simulink model "Model_FC_v16_Edit_for_Full_Scale_Fuel_Cell_GAS"  (R2018a)
settings: Solver=VariableStepAuto  StartTime=0  StopTime=inf  FixedStep=0.01  RelTol=1e-3  EnableMultiTasking=on
undefined symbols (not defined in the file): sigbuilder_block
libraries: fl_lib x8, simulink x6, nesl_utility x4, autolibdcdc x1, powerlib x1
(part 1 of 3)
settings Model: SimulationMode=accelerator  Creator=Mina  LastModifiedBy=Mina
settings SolverCC: ZeroCrossControl=EnableAll  ZeroCrossAlgorithm=Adaptive
settings DataIOCC: LimitDataPoints=on  SaveFormat=Array
settings OptimizationCC: BlockReduction=off  ConditionallyExecuteInputs=off  EfficientMapNaN2IntZero=off  LifeSpan=inf  SimCompilerOptimization=on  AccelVerboseBuild=on
settings DebuggingCC: IgnoredZcDiagnostic=none  SFUnexpectedBacktrackingDiag=warning  SFNoUnconditionalDefaultTransitionDiag=warning  SFExecutionAtInitializationDiag=none
settings HardwareCC: ProdBitPerPointer=32  ProdBitPerSizeT=32  ProdBitPerPtrDiffT=32  ProdLargestAtomicFloat=None  ProdIntDivRoundTo=Undefined  ProdEndianess=Unspecified  ProdWordSize=32  ProdHWDeviceType=32-bit Generic  TargetBitPerPointer=64  TargetBitPerSizeT=64  TargetBitPerPtrDiffT=64  TargetLongLongMode=on  TargetIntDivRoundTo=Zero  TargetEndianess=LittleEndian  TargetWordSize=64  TargetHWDeviceType=MATLAB Host  ProdEqTarget=off
settings ModelReferenceCC: PropagateSignalLabelsOutOfModel=off
settings CodeAppCC: MaxIdLength=128  StateflowObjectComments=on
settings GRTTargetCC: TargetLangStandard=C89/C90 (ANSI)  CombineOutputUpdateFcns=off  GRTInterface=on
settings ConfigComp: CovMetricSettings=dw  CovHtmlReporting=on  CovSaveCumulativeToWorkspaceVar=on  CovSaveSingleToWorkspaceVar=on  CovExternalEMLEnable=off
settings SimscapeCC: SimscapeNormalizeSystem=off

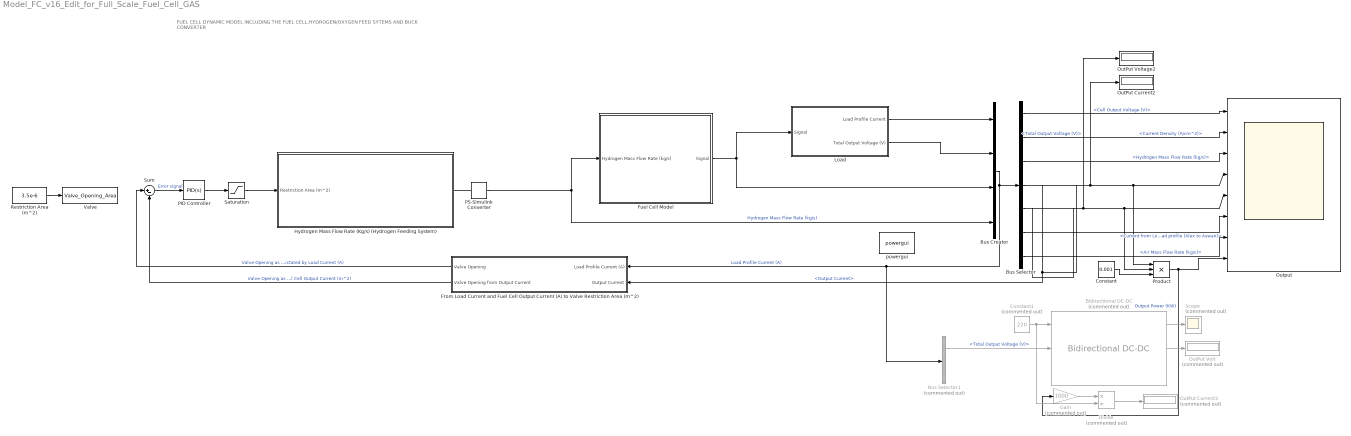
== system Model_FC_v16_Edit_for_Full_Scale_Fuel_Cell_GAS ==
  note: FUEL CELL DYNAMIC MODEL INCLUDING THE FUEL CELL,HYDROGEN/OXYGEN FEED SYTEMS AND BUCK CONVERTER
  Bidirectional DC-DC : autolibdcdc/Bidirectional DC-DC  Commented=on  Tc=1/1000  Vinit=0  Plimit=100000  param_loss=Single efficiency measurement  eff=98  v_loss_bp=[0 200 400 600 800 1000]  i_loss_bp=[0 25 50 75 100]  losses_table=[100 100 100 100 100;100 150 200 250 300;100 200 300 400 500;100 250 400 550 700;100 300 500 700 900;100 350 600 850 1100]  v_eff_bp=[200 400 600 800 1000]  i_eff_bp=[25 50 75 100]  efficiency_table=[96.2 98.1 98.7 99;98.1 99 99.4 99.5;98.7 99.4 99.6 99.7;99 99.5 99.7 99.8;99.2 99.6 99.7 99.8]  x_v_bp=[-1000 -800 -600 -400 -200 200 400 600 800 1000]  x_i_bp=[-100 -75 -50 -25 25 50 75 100]  x_losses_mat=[200.400801603196 225.67703109328 200.803212851408 201.612903225806 199.999999999997 200 225 200;160.320641282556 180.541624874624 201.005025125625 202.020202020203 200 200 180 160;180.541624874624 180.722891566267 181.086519114686 197.568389057748 194.999999999999 179.999999999997 180 180;201.005025125625 181.086519114686 202.020202020203 193.67991845056 190 200 179.999999999997 200;202.020202020203 197.568389057748 193.67991845056 197.505197505197 190 190 194.999999999999 200;200 194.999999999999 190 190 197.505197505197 193.67991845056 197.568389057748 202.020202020203;200 179.999999999997 200 190 193.67991845056 202.020202020203 181.086519114686 201.005025125625;180 180 179.999999999997 194.999999999999 197.568389057748 181.086519114686 180.722891566267 180.541624874624;160 180 200 200 202.020202020203 201.005025125625 180.541624874624 160.320641282556;200 225 200 199.999999999997 201.612903225806 200.803212851408 225.67703109328 200.400801603196]
      settings: SourceProductName=Powertrain Blockset  SourceProductBaseCode=PW
  Bus Creator : BusCreator  Inputs=4
  Bus Selector : BusSelector  OutputSignals=signal3.Cell Output Voltage (V),signal3.Current Density (A/cm^2),Hydrogen Mass Flow Rate (kg/s),signal3.Output Current,Total Output Voltage (V),Current from Load profile (Alex to Aswan),signal3.Air Mass Flow Rate (kg/s)
  Bus Selector1 : BusSelector  Commented=on  OutputSignals=Total Output Voltage (V),signal3.Output Current
  Constant : Constant  Value=0.001
  Constant1 : Constant  Commented=on  Value=220
  Divide : Product  Commented=on  Inputs=*/
  From Load Current and Fuel Cell Output Current (A) to Valve Restriction Area (m^2) : Subsystem
  Fuel Cell Model : Subsystem  mask(Fuel Cell Model){Temperature_c=80, Hydrogen_Pressure_atm=8, Air_Pressure_atm=8, Number_of_cells=208, Cell_Area_cm_squared=4397.14, Alpha_charge_Transfer_Coefficient=0.5, Exchange_Current_Density_i0=0.00000012246, Internal_Resistance_r=0.019, Amplification_Constant_Alpha1=0.085, Limiting_Current_Density_i_l=2, Mass_Transport_Limit_k=1.1, Dynamic_Response=[5 1]}
      mask prompts: Temperature_c "Temperature (c)"; Hydrogen_Pressure_atm "Hydrogen Pressure (atm)"; Air_Pressure_atm "Air Pressure (atm)"; Number_of_cells "Number Of Cells"; Cell_Area_cm_squared "Cell Area (cm^2)"; Alpha_charge_Transfer_Coefficient "Alpha (Charge Transfer Coefficient)"; Exchange_Current_Density_i0 "Exchange Current Density (i_0)(A/cm^2)"; Internal_Resistance_r "Internal Resistance (r)(Ohm)"; Amplification_Constant_Alpha1 "Amplification Constant (Alpha1)"; Limiting_Current_Density_i_l "Limiting Current Density (i_L)(A/cm^2)"; Mass_Transport_Limit_k "Mass Transport Limit (k)"; Dynamic_Response "Cell Dynamic Response (s)"
      mask help:
      | This is a mathematical Fuel Cell dynamic model. It operates under the Following Assumptions:
      | 1-The model is dynamic ,ie, it models the fuel cell behavior with respect to time.
      | 2-Fuel Cell Temperature is Constant.
      | 3-No Excess Hydrogen ,ie, Every Hydrogen molecule that enters the fuel cell Stack reacts to produce electricity.
      | 4-No excess Air.
      | 5-Concentration Losses are not calculated in the Model as we will never approach this region during operation.
      mask TypeOptions Temperature_c:
      | Stack Temperature
      | (C)/Value
      mask TypeOptions Hydrogen_Pressure_atm: Hydrogen Pressure (atm)/Value
      mask TypeOptions Air_Pressure_atm: Air Pressue (atm)/Value
      mask TypeOptions Number_of_cells: Number of Cells/Value
      mask TypeOptions Cell_Area_cm_squared:
      | Cell Area
      | (cm^2)/Value
      mask TypeOptions Alpha_charge_Transfer_Coefficient:
      | From Current Density (A//cm^2)
      | To
      | Overvoltages (V)/Activation Overvoltage/Alpha
      | Charge Transfer Coefficient1/Value
      mask TypeOptions Exchange_Current_Density_i0:
      | From Current Density (A//cm^2)
      | To
      | Overvoltages (V)/Activation Overvoltage/Reference Exchange Current Density
      | (I_0)1/Value
      mask TypeOptions Internal_Resistance_r:
      | From Current Density (A//cm^2)
      | To
      | Overvoltages (V)/Ohmic Overvoltage/Internal Resistance
      | (r)/Value
      mask TypeOptions Amplification_Constant_Alpha1:
      | From Current Density (A//cm^2)
      | To
      | Overvoltages (V)/Concentration Overvoltage/Amplification Constant
      | Alpha2/Value
      mask TypeOptions Limiting_Current_Density_i_l:
      | From Current Density (A//cm^2)
      | To
      | Overvoltages (V)/Concentration Overvoltage/Limiting Current
      | (i_L)1/Value
      mask TypeOptions Mass_Transport_Limit_k:
      | From Current Density (A//cm^2)
      | To
      | Overvoltages (V)/Concentration Overvoltage/Mass Transport Constant
      | (K)1/Value
      mask TypeOptions Dynamic_Response: Cell dynamic/Denominator
      mask DialogControl Operating_Conditions Prompt: Operating Conditions
      mask DialogControl Fuel_Cell_Parameters Prompt: Fuel Cell Parameters
      mask Display: image(imread('power_fuelcell.png'));port_label('output',1,'m');
  Gain : Gain  Commented=on  Gain=1000
  Hydrogen Mass Flow Rate (Kg/s) (Hydrogen Feeding System) : Subsystem
  Load : Subsystem
  OutPut Current2 : Display
  OutPut Current3 : Display  Commented=on
  OutPut Volt : Display  Commented=on
  OutPut Voltage2 : Display
  "Output " : Scope  NumInputPorts=8
  PID Controller : simulink/Continuous/PID Controller  Controller=PID  TimeDomain=Continuous-time  SampleTime=-1  IntegratorMethod=Forward Euler  FilterMethod=Forward Euler  Form=Parallel  UseFilter=on  ControllerParametersSource=internal  P=0.5  I=0.7  D=0.01  N=100  InitialConditionSource=internal  InitialConditionForIntegrator=0  InitialConditionForFilter=0  ExternalReset=none  LimitOutput=on  UpperSaturationLimit=1.5e-5  LowerSaturationLimit=-inf  LinearizeAsGain=on  AntiWindupMode=none  Kb=1  TrackingMode=off  Kt=1  PParamMin=[]  PParamMax=[]  IParamMin=[]  IParamMax=[]  DParamMin=[]  DParamMax=[]  NParamMin=[]  NParamMax=[]  KbParamMin=[]  KbParamMax=[]  KtParamMin=[]  KtParamMax=[]  POutMin=[]  POutMax=[]  IOutMin=[]  IOutMax=[]  DOutMin=[]  DOutMax=[]  NOutMin=[]  NOutMax=[]  KbOutMin=[]  KbOutMax=[]  KtOutMin=[]  KtOutMax=[]  IntegratorOutMin=[]  IntegratorOutMax=[]  FilterOutMin=[]  FilterOutMax=[]  SumOutMin=[]  SumOutMax=[]  SumI1OutMin=[]  SumI1OutMax=[]  SumI2OutMin=[]  SumI2OutMax=[]  SumI3OutMin=[]  SumI3OutMax=[]  SumDOutMin=[]  SumDOutMax=[]  SaturationOutMin=[]  SaturationOutMax=[]  IntegratorContinuousStateAttributes=''  IntegratorStateMustResolveToSignalObject=off  IntegratorRTWStateStorageClass=Auto  FilterContinuousStateAttributes=''  FilterStateMustResolveToSignalObject=off  FilterRTWStateStorageClass=Auto  DifferentiatorICPrevScaledInput=0  DifferentiatorOutMin=[]  DifferentiatorOutMax=[]  InitialConditionSetting=State (most efficient)  FilterDiffOutCoefMin=[]  FilterDiffOutCoefMax=[]  SumDenOutMin=[]  SumDenOutMax=[]  SumNumOutMin=[]  SumNumOutMax=[]  ReciprocalOutMin=[]  ReciprocalOutMax=[]  DivideOutMin=[]  DivideOutMax=[]  TunerSelectOption=Transfer Function Based (PID Tuner App)
  PS-Simulink Converter : nesl_utility/PS-Simulink Converter  PhysicalDomain=network_engine_domain  SubClassName=ps_output  LeftPortType=input  RightPortType=output  PseudoPeriodic=off  Frequencies=[]  Unit=1  AffineConversion=off
  Product : Product  Inputs=3
  "Restriction Area (m^2) " : Constant  Value=3.5e-6  VectorParams1D=off
  Saturation : Saturate  UpperLimit=2.7e-5  LowerLimit=0
  Scope : Scope  Commented=on
  Sum : Sum  Inputs=|+-
  Valve : ToWorkspace  VariableName=Valve_Opening_Area  SaveFormat=Timeseries  SampleTime=-1
  powergui : powerlib/powergui  Priority=1  SimulationMode=Discrete  SampleTime=50e-6  frequency=60  Iterations=50  frequencyindice=0  Pbase=100e6  ErrMax=1e-4  UnitsV=kV  UnitsW=MW  buscounter=0  FunctionMessages=off  echomessages=off  EnableUseOfTLC=off  CurrentSourceSwitches=off  DisableSnubberDevices=off  DisableRonSwitches=off  DisableVfSwitches=off  DisplayEquations=off  SolverType=Tustin/Backward Euler (TBE)  Interpol=off  ExternalGateDelay=off  methode=off  Ts=100  x0status=blocks  SPID=off  SwTol=0  HookPort=off  RestoreLinks=warning  ResistiveCurrentMeasurement=off  Frange=[0:2:500]  Ylog=off  Xlog=on  ShowGrid=off  save=off  variable=ZData  structure=0  ZoomFFT=off  StartTime=0.0  cycles=1  DisplayStyle=1  fundamental=60  FreqAxis=off  MaxFrequency=1000  frequencyindicesteady=1  RmsSteady=1  display=off
  wires:
  Fuel Cell Model/1(Signal) -> Bus Creator/3, Load/1(Signal)
  PS-Simulink Converter/1 -> Fuel Cell Model/1(Hydrogen Mass Flow Rate (kg/s)), Bus Creator/4  "Hydrogen Mass Flow Rate (kg/s)"
  Load/1(Load Profile Current) -> Bus Creator/1
  Load/2(Total Output Voltage (V)) -> Bus Creator/2
  Bus Selector/1 -> "Output "/1  "<Cell Output Voltage (V)>"
  Bus Selector/2 -> "Output "/2  "<Current Density (A/cm^2)>"
  Bus Selector/3 -> "Output "/3  "<Hydrogen Mass Flow Rate (kg/s)>"
  Bus Selector/4 -> OutPut Current2/1, Product/1, "Output "/4, From Load Current and Fuel Cell Output Current (A) to Valve Restriction Area (m^2)/2(Output Current)  "<Output Current>"
  Bus Selector/5 -> OutPut Voltage2/1, Product/2, "Output "/5  "<Total Output Voltage (V)>"
  From Load Current and Fuel Cell Output Current (A) to Valve Restriction Area (m^2)/1(Valve Opening) -> Sum/1  "Valve Opening as dictated by Load Current (A)"
  "Restriction Area (m^2) "/1 -> Valve/1
  From Load Current and Fuel Cell Output Current (A) to Valve Restriction Area (m^2)/2(Valve Opening from Output Current) -> Sum/2  "Valve Opening as dictated by Fuel Cell Output Current (m^2)"
  Sum/1 -> PID Controller/1  "Error signal"
  Bus Creator/1 -> From Load Current and Fuel Cell Output Current (A) to Valve Restriction Area (m^2)/1(Load Profile Current (A)), Bus Selector1/1, Bus Selector/1  "Load Profile Current (A)"
  Bus Selector/6 -> "Output "/6  "<Current from Load profile (Alex to Aswan)>"
  PID Controller/1 -> Saturation/1
  Saturation/1 -> Hydrogen Mass Flow Rate (Kg/s) (Hydrogen Feeding System)/1(Restriction Area (m^2))
  Bus Selector/7 -> "Output "/7  "<Air Mass Flow Rate (kg/s)>"
  Product/1 -> Gain/1, "Output "/8  "Output Power (KW)"
  Constant/1 -> Product/3
  Constant1/1 -> Divide/2, Bidirectional DC-DC/1
  Bidirectional DC-DC/1 -> Scope/1
  Bidirectional DC-DC/2 -> OutPut Volt/1
  Bus Selector1/1 -> Bidirectional DC-DC/2  "<Total Output Voltage (V)>"
  Divide/1 -> OutPut Current3/1
  Gain/1 -> Divide/1
  connections:
  PS-Simulink Converter/LConn1 -- Hydrogen Mass Flow Rate (Kg/s) (Hydrogen Feeding System)/RConn1

== system Model_FC_v16_Edit_for_Full_Scale_Fuel_Cell_GAS/From Load Current and Fuel Cell Output Current (A) to Valve Restriction Area (m^2) ==
  note: (3.0735e-14*(u(1)^3)) + (-5.0428e-11*(u(1)^2)) +(4.1772e-08*u(1)) + 2.7105e-07
  note: FEEDBACK BLOCK
  note: This block is the feedback block that controls the Flow control valve of the Hydrogen feeding system
      | I NPUTS: A) load Current (A) OUTPUTS: A) valve Restriction Area(m^2) as dictated by the Load Current
      | B) Output Current of the Fuel Cell (A) B) valve Restriction Area (m^2) as dictated by the Fuel Cell output current
  Load Profile Current (A) : Inport
  Output Current : Inport  Port=2
  Subsystem : Subsystem
  Subsystem1 : Subsystem
  Valve Opening : Outport
  Valve Opening from Output Current : Outport  Port=2
  wires:
  Output Current/1 -> Subsystem/1(In1)
  Subsystem/1(Valve Opening from Output Current) -> Valve Opening from Output Current/1
  Load Profile Current (A)/1 -> Subsystem1/1(In1)
  Subsystem1/1(Out1) -> Valve Opening/1

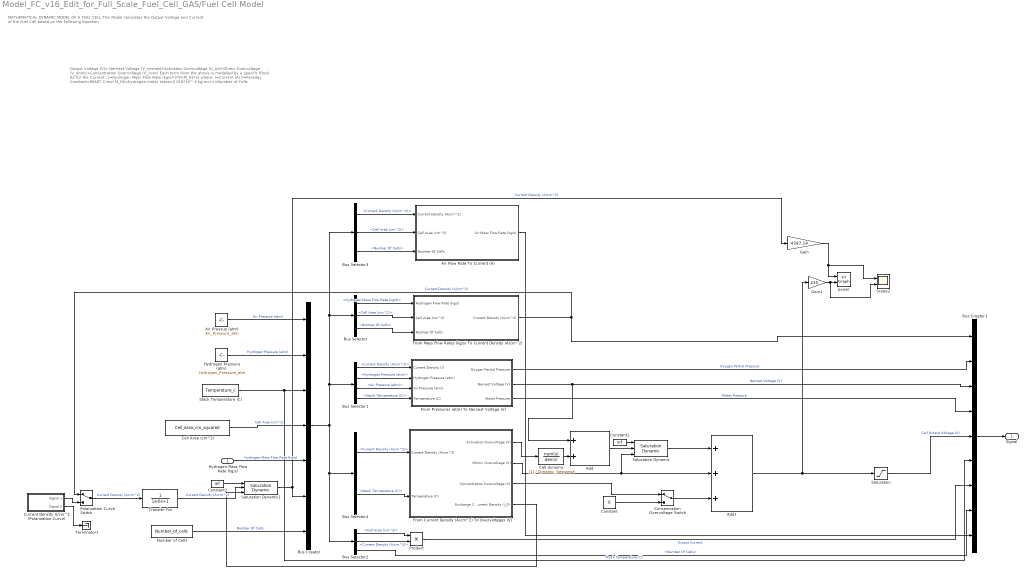
== system Model_FC_v16_Edit_for_Full_Scale_Fuel_Cell_GAS/Fuel Cell Model ==
  note: Output Voltage (V)= Nernest Voltage (V_nernest)-Activation Overvoltage (V_Act)-Ohmic Overvoltage (V_ohmic)-Concentration Overvoltage (V_conc)
      | Each term from the above is modelled by a specific Block.
      | As for the Current :
      |
      | I=Hydrogen Mass Flow Rate (kg/s)*2*F/(M_H2*n)
      | where: I=Current (A)
      | F=Faraday Constant=96487 C/mol
      | M_H2=hydrogen molar mass=2.016*10^-3 kg/mol
      | n=Number of Cells
  note: MATHEMATICAL DYNAMIC MODEL OF A FUEL CELL
      | This Model calculates the Output Voltage and Current of the Fuel Cell based on the Following Equation
  Hydrogen Mass Flow Rate (kg/s) : Inport
  " From Current Density (A/cm^2) To Overvoltages (V)" : Subsystem
  Add : Sum
  Add1 : Sum  Inputs=+++
  Air Flow Rate To Current (A) : Subsystem
  Air Pressue (atm) : Constant  Value=Air_Pressure_atm
  Bus Creator : BusCreator  Inputs=7
  Bus Creator1 : BusCreator  Inputs=9
  Bus Selector : BusSelector  OutputSignals=Hydrogen Mass Flow Rate (kg/s),Cell Area (cm^2),Number Of Cells
  Bus Selector1 : BusSelector  OutputSignals=Current Density (A/cm^2),Hydrogen Pressure (atm),Air Pressure (atm),Stack Temperature (C)
  Bus Selector2 : BusSelector  OutputSignals=Cell Area (cm^2),Current Density (A/cm^2),Number Of Cells
  Bus Selector3 : BusSelector  OutputSignals=Current Density (A/cm^2),Cell Area (cm^2),Number Of Cells
  Bus Selector4 : BusSelector  OutputSignals=Current Density (A/cm^2),Stack Temperature (C)
  Cell Area (cm^2) : Constant  Value=Cell_Area_cm_squared
  Cell dynamic : TransferFcn  Denominator=Dynamic_Response
  Concentration Overvoltage Switch : ManualSwitch
  Constant : Constant  Value=0
  Constant1 : Constant  Value=inf
  Constant2 : Constant  Value=inf
  Current Density A/cm^2 (Polarization Curve) : Subsystem  Tag=STV Subsys  LoadFcn=sigbuilder_block('load');  StartFcn=sigbuilder_block('start');  StopFcn=sigbuilder_block('stop');  ClipboardFcn=sigbuilder_block('clipboard');  mask(Sigbuilder block){tuvar=[0:10]}
      mask help: Simulink:masks:SigbuilderBlock_MD
      mask init:
      | if ~strcmp(get_param(bdroot(gcbh),'SimulationStatus'),'stopped') tuvar = sigbuilder_block('maskInit'); end
      settings: CopyFcn=sigbuilder_block('copy');  DeleteFcn=sigbuilder_block('delete');  ModelCloseFcn=sigbuilder_block('modelClose');  PreSaveFcn=sigbuilder_block('preSave');  PauseFcn=sigbuilder_block('pause');  ContinueFcn=sigbuilder_block('continue');  NameChangeFcn=sigbuilder_block('namechange');  OpenFcn=sigbuilder_block('open',[403.5 117 550.5 359.25 ]);  CloseFcn=sigbuilder_block('close');
      mask Display: plot(0, 0, 100, 100,[2, 2, 32, 32, 2], [68, 8, 8, 68, 68],[32, 2], [38, 38], [32, 19, 2],[53, 60, 44], [32, 17, 17, 2],[16, 16, 31, 31]);txt = getActiveGroup(gcbh);text(2, 100, txt,'verticalAlignment', 'top');
  From Mass Flow Rates (kg/s) To Current Density (A/cm^2) : Subsystem
  From Pressures (atm) To Nernest Voltage (V) : Subsystem
  Gain : Gain  Gain=4397.14
  Gain1 : Gain  Gain=235
  Hydrogen Pressure (atm) : Constant  Value=Hydrogen_Pressure_atm
  Number of Cells : Constant  Value=Number_of_cells
  Polarization Curve Switch : ManualSwitch
  Product : Product
  Saturation : Saturate  UpperLimit=inf  LowerLimit=0  ZeroCross=off
  Saturation Dynamic : simulink/Discontinuities/Saturation Dynamic  OutMin=[]  OutMax=[]  OutDataTypeStr=Inherit: Same as second input  OutDataType=sfix(16)  OutScaling=2^-10  DoSatur=off
  Saturation Dynamic1 : simulink/Discontinuities/Saturation Dynamic  OutMin=[]  OutMax=[]  OutDataTypeStr=Inherit: Same as second input  OutDataType=sfix(16)  OutScaling=2^-10  DoSatur=off
  Scope2 : Scope  NumInputPorts=2
  Stack Temperature (C) : Constant  Value=Temperature_c
  Terminator1 : Terminator
  Transfer Fcn : TransferFcn  Denominator=[1e-6 1]
  power : simulink/Sinks/XY Graph  xmin=0  xmax=20  ymin=0.0  ymax=20  st=0
  Signal : Outport
  wires:
  Saturation/1 -> Bus Creator1/5  "Cell Output Voltage (V)"
  Current Density A/cm^2 (Polarization Curve)/1(Signal 1) -> Polarization Curve Switch/2
  Hydrogen Mass Flow Rate (kg/s)/1 -> Bus Creator/5  "Hydrogen Mass Flow Rate (kg/s)"
  Bus Creator/1 -> Bus Selector2/1, Bus Selector4/1, Bus Selector1/1, Bus Selector3/1, Bus Selector/1
  From Mass Flow Rates (kg/s) To Current Density (A/cm^2)/1(Current Density (A/cm^2)) -> Bus Creator1/1, Polarization Curve Switch/1  "Current Density (A/cm^2)"
  Bus Selector/1 -> From Mass Flow Rates (kg/s) To Current Density (A/cm^2)/1(Hydrogen Flow Rate (kg/s))  "<Hydrogen Mass Flow Rate (kg/s)>"
  Bus Selector/2 -> From Mass Flow Rates (kg/s) To Current Density (A/cm^2)/2(Cell Area (cm^2))  "<Cell Area (cm^2)>"
  From Pressures (atm) To Nernest Voltage (V)/2(Nernest Voltage (V)) -> Bus Creator1/3, Add/1  "Nernest Voltage (V)"
  Bus Selector1/1 -> From Pressures (atm) To Nernest Voltage (V)/1(Current Density (i))  "<Current Density (A/cm^2)>"
  Bus Selector1/2 -> From Pressures (atm) To Nernest Voltage (V)/2(Hydrogen Pressure (atm))  "<Hydrogen Pressure (atm)>"
  Bus Selector1/3 -> From Pressures (atm) To Nernest Voltage (V)/3(Air Pressure (atm))  "<Air Pressure (atm)>"
  Bus Selector1/4 -> From Pressures (atm) To Nernest Voltage (V)/4(Temperature (C))  "<Stack Temperature (C)>"
  From Pressures (atm) To Nernest Voltage (V)/1(Oxygen Partial Pressure) -> Bus Creator1/2  "Oxygen Partial Pressure"
  From Pressures (atm) To Nernest Voltage (V)/3(Water Pressure) -> Bus Creator1/4  "Water Pressure"
  Bus Selector4/1 -> " From Current Density (A/cm^2) To Overvoltages (V)"/1(Current Density (A/cm^2))  "<Current Density (A/cm^2)>"
  Bus Selector4/2 -> " From Current Density (A/cm^2) To Overvoltages (V)"/2(Temperature (C))  "<Stack Temperature (C)>"
  " From Current Density (A/cm^2) To Overvoltages (V)"/1(Activation Overvoltage (V)) -> Cell dynamic/1
  Bus Creator1/1 -> Signal/1
  Polarization Curve Switch/1 -> Transfer Fcn/1  "Current Density (A/cm^2)"
  Constant2/1 -> Saturation Dynamic1/1
  " From Current Density (A/cm^2) To Overvoltages (V)"/4(Exchange Current Density (i_0)) -> Saturation Dynamic1/3
  Add1/1 -> Gain1/1, Saturation/1
  Cell dynamic/1 -> Add/2
  Add/1 -> Saturation Dynamic/2
  Constant1/1 -> Saturation Dynamic/1
  Saturation Dynamic/1 -> Add1/1
  " From Current Density (A/cm^2) To Overvoltages (V)"/3(Concentration Overvoltage (V)) -> Concentration Overvoltage Switch/1
  Bus Selector2/2 -> Product/2  "<Current Density (A/cm^2)>"
  Bus Selector2/1 -> Product/1  "<Cell Area (cm^2)>"
  Product/1 -> Bus Creator1/7  "Output Current"
  Bus Selector/3 -> From Mass Flow Rates (kg/s) To Current Density (A/cm^2)/3(Number Of Cells)  "<Number Of Cells>"
  Bus Selector2/3 -> Bus Creator1/8  "<Number Of Cells>"
  Saturation Dynamic1/1 -> Bus Creator/6, Gain/1  "Current Density (A/cm^2)"
  Transfer Fcn/1 -> Saturation Dynamic1/2  "Current Density (A/cm^2)"
  Stack Temperature (C)/1 -> Bus Creator/3, Bus Creator1/6  "Stack Temperature (C)"
  Hydrogen Pressure (atm)/1 -> Bus Creator/2  "Hydrogen Pressure (atm)"
  Air Pressue (atm)/1 -> Bus Creator/1  "Air Pressure (atm)"
  Number of Cells/1 -> Bus Creator/7  "Number Of Cells"
  Cell Area (cm^2)/1 -> Bus Creator/4  "Cell Area (cm^2)"
  " From Current Density (A/cm^2) To Overvoltages (V)"/2(Ohmic Overvoltage (V)) -> Saturation Dynamic/3, Add1/2
  Concentration Overvoltage Switch/1 -> Add1/3
  Constant/1 -> Concentration Overvoltage Switch/2
  Air Flow Rate To Current (A)/1(Air Mass Flow Rate (kg/s)) -> Bus Creator1/9
  Current Density A/cm^2 (Polarization Curve)/2(Signal 2) -> Terminator1/1
  Gain/1 -> Scope2/1, power/1
  Gain1/1 -> Scope2/2, power/2
  Bus Selector3/1 -> Air Flow Rate To Current (A)/1(Current Density (A/cm^2))  "<Current Density (A/cm^2)>"
  Bus Selector3/2 -> Air Flow Rate To Current (A)/2(Cell Area (cm^2))  "<Cell Area (cm^2)>"
  Bus Selector3/3 -> Air Flow Rate To Current (A)/3(Number Of Cells)  "<Number Of Cells>"
